simulink model "ModelosPlanta"  (R2024b)
settings: Solver=VariableStepAuto  StartTime=0.0  StopTime=10  RelTol=1e-3
values from neighbouring files (symbols this model uses):
  A = Lm / I    (= 19.8203592814)    [Grafico_comparacion_controlador_continuo_discreto.m]    (also in Grafico_comparacion_modelo_linealizado.m = -C * sin(theta_eq) / I; PIDf_Asignacion_Polos.m; SimulacionModelosMallaCerradaConControlador.m; Variables_sistema_para_simulink.m)
  angulo_equilibrio = 10 * (pi/180)    (= 0.174532925199)    [Grafico_comparacion_controlador_continuo_discreto.m]    (also in Obtener_modelo_motor.m = 0; PIDf_Asignacion_Polos.m = 0; SimulacionModelosMallaCerradaConControlador.m = i * (pi/180); Variables_sistema_para_simulink.m = 0)
  B = C * sin(angulo_equilibrio) / I    [Grafico_comparacion_controlador_continuo_discreto.m]    (also in Grafico_comparacion_modelo_linealizado.m = 19.8203592814; PIDf_Asignacion_Polos.m; SimulacionModelosMallaCerradaConControlador.m; Variables_sistema_para_simulink.m)
  C = Pcp * Lcp + Pv1 * Lv1 - Pc * Lc - Pv2 * Lv2 - Pj * Lj - Pm * Lm    (= -0.1326097161)    [Constantes_helicoptero.m]    (also in Grafica_PWMvsFuerza_equilibrio.m = -0.1326; Grafica_validacion_superpuestas.m = -0.1326; Grafico_comparacion_controlador_continuo_discreto.m = -0.1326; Grafico_comparacion_modelo_linealizado.m = -0.1326)
  condicion_inicial_angulo_modelo_no_lineal = angulo_equilibrio    (= 0.174532925199)    [Grafico_comparacion_controlador_continuo_discreto.m]    (also in SimulacionModelosMallaCerradaConControlador.m = angulo_equilibrio)
  fuerza_equilibrio = -(C * cos(angulo_equilibrio)) / Lm    [Grafico_comparacion_controlador_continuo_discreto.m]    (also in SimulacionModelosMallaCerradaConControlador.m)
  I = Icp + Im + Ij + Iv1 + Iv2 + Ic    (= 0.0166790788666)    [Constantes_helicoptero.m]    (also in Grafica_PWMvsFuerza_equilibrio.m = 0.0167; Grafica_validacion_superpuestas.m = 0.0167; Grafico_comparacion_controlador_continuo_discreto.m = 0.0167; Grafico_comparacion_modelo_linealizado.m = 0.0167)
  Lm = 2 * Lv2 + 0.014    (= 0.331)    [Constantes_helicoptero.m]    (also in Grafica_PWMvsFuerza_equilibrio.m; Grafica_validacion_superpuestas.m = 0.35; Grafico_comparacion_controlador_continuo_discreto.m; Grafico_comparacion_modelo_linealizado.m)
  m = 0.001586    [Grafica_PWMvsFuerza_equilibrio.m]    (also in Grafico_comparacion_controlador_continuo_discreto.m; Obtener_modelo_motor.m = coeficientes(1); PIDf_Asignacion_Polos.m; SimulacionModelosMallaCerradaConControlador.m)
  PWM_equilibrio = (fuerza_equilibrio-r)/m    [Grafico_comparacion_controlador_continuo_discreto.m]    (also in SimulacionModelosMallaCerradaConControlador.m = (fuerza_equilibrio - r) / m)
  r = -1.597768    [Grafica_PWMvsFuerza_equilibrio.m]    (also in Grafico_comparacion_controlador_continuo_discreto.m = -1.692631; Obtener_modelo_motor.m = coeficientes(2); SimulacionModelosMallaCerradaConControlador.m)
libraries: slpidlib x1
settings Model: Creator=UTEC-5695  LastModifiedBy=lucas

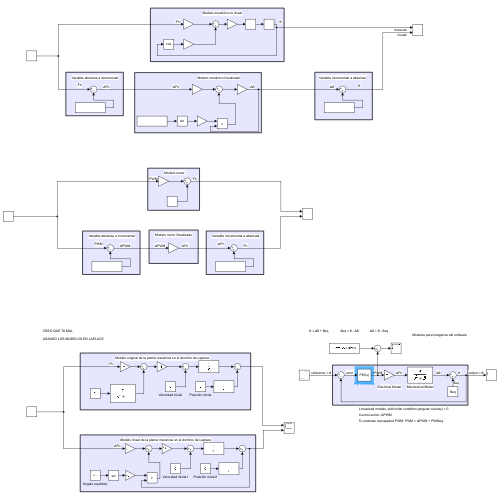
[thumbnail: Simulink's stored preview of the top-level diagram]
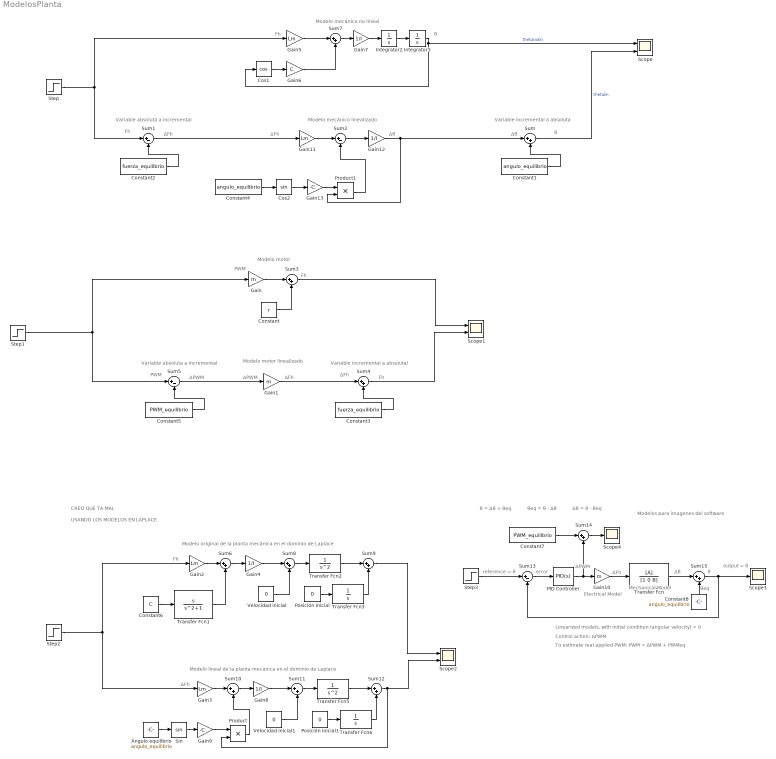
== system ModelosPlanta ==
  note: Modelos para imagenes del software
  note: Modelo original de la planta mecánica en el dominio de Laplace
  note: Fh
  note: USANDO LOS MODELOS EN LAPLACE
  note: CREO QUE TA MAL
  note: Variable absoluta a incremental
  note: θ
  note: Modelo mecánico linealizado
  note: Modelo mecánico no lineal
  note: ΔFh
  note: Fh
  note: Δθ
  note: Δθ
  note: θ
  note: ΔFh
  note: Fh
  note: Variable incremental a absoluta
  note: Modelo motor
  note: PWM
  note: Fh
  note: Modelo motor linealizado
  note: ΔPWM
  note: ΔFh
  note: Fh
  note: ΔFh
  note: Variable incremental a absolutal
  note: Variable absoluta a incremental
  note: PWM
  note: ΔPWM
  note: Modelo lineal de la planta mecánica en el dominio de Laplace
  note: ΔFh
  note: ΔFh
  note: Δθ
  note: ΔPWM
  note: error
  note: reference = θ
  note: Δθ = θ - θeq
  note: θeq = θ - Δθ
  note: θeq
  note: θ = Δθ + θeq
  note: output = θ
  note: Linearized models, with initial condition (angular velocity) = 0
  note: Mechanical Model
  note: Electrical Model
  note: To estimate real applied PWM: PWM = ΔPWM + PWMeq
  note: Control action: ΔPWM
  note: θ
  Constant : Constant  Value=r
  Constant1 : Constant  Value=angulo_equilibrio
  Constant2 : Constant  Value=fuerza_equilibrio
  Constant3 : Constant  Value=fuerza_equilibrio
  Constant4 : Constant  Value=angulo_equilibrio
  Constant5 : Constant  Value=PWM_equilibrio
  Constant6 : Constant  Value=C
  Constant7 : Constant  Value=PWM_equilibrio
  Constant8 : Constant  Value=angulo_equilibrio
      mask Display: disp('θeq');
  Cos1 : Trigonometry  Operator=cos
  Cos2 : Trigonometry
  Gain : Gain  Gain=m
  Gain1 : Gain  Gain=m
  Gain10 : Gain  Gain=m
  Gain{2..3,5,11} (4 alike) : Gain  Gain=Lm
  Gain{4,7..8,12} (4 alike) : Gain  Gain=1/I
  Gain13 : Gain  Gain=-C
  Gain6 : Gain  Gain=C
  Gain9 : Gain  Gain=-C
  Integrator2 : Integrator
  Integrator3 : Integrator  InitialCondition=condicion_inicial_angulo_modelo_no_lineal
  PID Controller : slpidlib/PID Controller  Controller=PID  Form=Parallel  TimeDomain=Continuous-time  UseExternalTs=off  SampleTime=-1  IntegratorMethod=Forward Euler  FilterMethod=Forward Euler  ControllerParametersSource=internal  P=5.90675147843486  I=0.276523260816653  UseKiTs=off  D=30.981969104075  UseExternalDerivativeSource=off  N=5.45397025421619  UseFilter=on  TunerSelectOption=Transfer Function Based (PID Tuner App)  InitialConditionSource=internal  InitialConditionForIntegrator=0  InitialConditionForFilter=0  DifferentiatorICPrevScaledInput=0  ExternalReset=none  TrackingMode=off  Kt=1  LimitOutput=off  SatLimitsSource=internal  UpperSaturationLimit=inf  LowerSaturationLimit=-inf  LinearizeAsGain=on  AntiWindupMode=none  Kb=1  LimitIntegrator=off  UpperIntegratorSaturationLimit=inf  LowerIntegratorSaturationLimit=-inf  POutMin=[]  POutMax=[]  IOutMin=[]  IOutMax=[]  DOutMin=[]  DOutMax=[]  NOutMin=[]  NOutMax=[]  SumOutMin=[]  SumOutMax=[]  SaturationOutMin=[]  SaturationOutMax=[]  PParamMin=[]  PParamMax=[]  IParamMin=[]  IParamMax=[]  DParamMin=[]  DParamMax=[]  NParamMin=[]  NParamMax=[]  KbParamMin=[]  KbParamMax=[]  KtParamMin=[]  KtParamMax=[]  KbOutMin=[]  KbOutMax=[]  KtOutMin=[]  KtOutMax=[]  IntegratorOutMin=[]  IntegratorOutMax=[]  FilterOutMin=[]  FilterOutMax=[]  SumI1OutMin=[]  SumI1OutMax=[]  SumI2OutMin=[]  SumI2OutMax=[]  SumI3OutMin=[]  SumI3OutMax=[]  SumI4OutMin=[]  SumI4OutMax=[]  SumDOutMin=[]  SumDOutMax=[]  DifferentiatorOutMin=[]  DifferentiatorOutMax=[]  FilterDiffOutCoefMin=[]  FilterDiffOutCoefMax=[]  ReciprocalOutMin=[]  ReciprocalOutMax=[]  SumDenOutMin=[]  SumDenOutMax=[]  SumNumOutMin=[]  SumNumOutMax=[]  DivideOutMin=[]  DivideOutMax=[]  UdiffTsProdOutMin=[]  UdiffTsProdOutMax=[]  NTsProdOutMin=[]  NTsProdOutMax=[]  UintegralTsProdOutMin=[]  UintegralTsProdOutMax=[]  UngainTsProdOutMin=[]  UngainTsProdOutMax=[]  ClampingZeroOutDataTypeStr=Inherit: Inherit via back propagation  ClampingZeroOutMin=[]  ClampingZeroOutMax=[]  FilterDenConstantOutDataTypeStr=Inherit: Inherit via back propagation  FilterDenConstantOutMin=[]  FilterDenConstantOutMax=[]  PCopyOutDataTypeStr=Inherit: Inherit via back propagation  PCopyOutMin=[]  PCopyOutMax=[]  NCopyOutDataTypeStr=Inherit: Inherit via back propagation  NCopyOutMin=[]  NCopyOutMax=[]  IntegratorContinuousStateAttributes=''  IntegratorStateMustResolveToSignalObject=off  IntegratorRTWStateStorageClass=Auto  FilterContinuousStateAttributes=''  FilterStateMustResolveToSignalObject=off  FilterRTWStateStorageClass=Auto  ParallelPVariant=InternalParameters  IdealPVariant=Disabled  IVariant=InternalParameters  DVariant=InternalParameters  IntegratorVariant=Continuous  SatVariant=Disabled  AWVariant=Passthrough  PCopyVariant=Disabled  TRVariant=Disabled  FdbkBlocksVariant=Forward  IdealPFdbkVariant=Disabled  SatFdbkVariant=Disabled  DerivativeFilterVariant=ContFilter  NVariant=InternalParameters  NCopyVariant=Disabled  FilterICVariant=InternalICsFilter  IntegratorICVariant=InternalICs  ExternalResetVariant=Disabled  TRSumVariant=Passthrough  SumFdbkVariant=Disabled  SumVariant=Sum_PID  TsampFilterVariant=InternalTs  TsampNgainVariant=Passthrough  TsampIntegralVariant=Disabled_SignalSpec  ExternalSaturationOutDataTypeStr=Inherit: Same as second input  DerivativeSourceVariant=ErrorSignal  PreIntVariant=InternalPreInt
  Posición inicial : Constant  Value=0
  Posición inicial1 : Constant  Value=0
  Product : Product
  Product1 : Product
  Scope : Scope  NumInputPorts=2
  Scope1 : Scope  NumInputPorts=2
  Scope2 : Scope  NumInputPorts=2
  Scope3 : Scope
  Scope4 : Scope
  Sin : Trigonometry
  Step : Step  Time=0  After=0  SampleTime=0
  Step1 : Step  After=1400  SampleTime=0
  Step2 : Step  After=0  SampleTime=0
  Step3 : Step  Time=0  After=0.2  SampleTime=0
  Sum{,3..4,6..12,14..15} (12 alike) : Sum  Inputs=|++
  Sum{1..2,5,13} (4 alike) : Sum  Inputs=|+-
  Transfer Fcn : TransferFcn  Numerator=[A]  Denominator=[1 0 B]
  Transfer Fcn1 : TransferFcn  Numerator=[1 0]  Denominator=[1 0 1]
  Transfer Fcn2 : TransferFcn  Denominator=[1 0 0]
  Transfer Fcn3 : TransferFcn  Denominator=[1 0]
  Transfer Fcn5 : TransferFcn  Denominator=[1 0 0]
  Transfer Fcn6 : TransferFcn  Denominator=[1 0]
  Velocidad inicial : Constant  Value=0
  Velocidad inicial1 : Constant  Value=0
  Ángulo equilibrio : Constant  Value=angulo_equilibrio
  wires:
  Sum7/1 -> Gain7/1
  Gain11/1 -> Sum2/1
  Constant4/1 -> Cos2/1
  Gain7/1 -> Integrator2/1
  Cos2/1 -> Gain13/1
  Gain6/1 -> Sum7/2
  Integrator3/1 -> Cos1/1, Scope/1  "thetanolin"
  Cos1/1 -> Gain6/1
  Integrator2/1 -> Integrator3/1
  Gain5/1 -> Sum7/1
  Sum2/1 -> Gain12/1
  Constant1/1 -> Sum/2
  Gain12/1 -> Sum/1, Product1/2
  Constant2/1 -> Sum1/2
  Step/1 -> Gain5/1, Sum1/1
  Sum1/1 -> Gain11/1
  Sum/1 -> Scope/2  "thetalin"
  Constant/1 -> Sum3/2
  Gain/1 -> Sum3/1
  Sum3/1 -> Scope1/1
  Step1/1 -> Gain/1, Sum5/1
  Sum5/1 -> Gain1/1
  Gain1/1 -> Sum4/1
  Constant3/1 -> Sum4/2
  Sum4/1 -> Scope1/2
  Constant5/1 -> Sum5/2
  Step2/1 -> Gain3/1, Gain2/1
  Gain2/1 -> Sum6/1
  Constant6/1 -> Transfer Fcn1/1
  Transfer Fcn1/1 -> Sum6/2
  Sum6/1 -> Gain4/1
  Gain4/1 -> Sum8/1
  Velocidad inicial/1 -> Sum8/2
  Sum8/1 -> Transfer Fcn2/1
  Transfer Fcn2/1 -> Sum9/1
  Transfer Fcn3/1 -> Sum9/2
  Posición inicial/1 -> Transfer Fcn3/1
  Sum11/1 -> Transfer Fcn5/1
  Transfer Fcn6/1 -> Sum12/2
  Gain3/1 -> Sum10/1
  Sum10/1 -> Gain8/1
  Velocidad inicial1/1 -> Sum11/2
  Transfer Fcn5/1 -> Sum12/1
  Gain8/1 -> Sum11/1
  Posición inicial1/1 -> Transfer Fcn6/1
  Sin/1 -> Gain9/1
  Ángulo equilibrio/1 -> Sin/1
  Gain9/1 -> Product/1
  Sum12/1 -> Scope2/2, Product/2
  Product/1 -> Sum10/2
  Sum9/1 -> Scope2/1
  Gain13/1 -> Product1/1
  Product1/1 -> Sum2/2
  Gain10/1 -> Transfer Fcn/1
  Transfer Fcn/1 -> Sum15/1
  Sum13/1 -> PID Controller/1
  PID Controller/1 -> Gain10/1, Sum14/2
  Step3/1 -> Sum13/1
  Sum15/1 -> Sum13/2, Scope3/1
  Constant8/1 -> Sum15/2
  Sum14/1 -> Scope4/1
  Constant7/1 -> Sum14/1
